simulink model "Gain_TestGen12"  (R2017b)
settings: Solver=FixedStepDiscrete  StartTime=0.0  StopTime=10.0  RelTol=1e-3
undefined symbols (not defined in the file): Block_TestLib, trigger
settings Model: Creator=ktrinh  LastModifiedBy=ktrinh
settings DebuggingCC: ParameterOverflowMsg=none

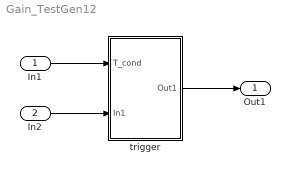
== system Gain_TestGen12 ==
  In1 : Inport
  In2 : Inport  Port=2
  trigger : Subsystem  AncestorBlock=Block_TestLib/trigger
  Out1 : Outport
  wires:
  In1/1 -> trigger/1(T_cond)
  In2/1 -> trigger/2(In1)
  trigger/1(Out1) -> Out1/1

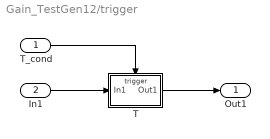
== system Gain_TestGen12/trigger ==
  T_cond : Inport  OutDataTypeStr=boolean
  In1 : Inport  Port=2
  T : Subsystem  TreatAsAtomicUnit=on
  Out1 : Outport
  wires:
  T_cond/1 -> T/Trigger
  In1/1 -> T/1(In1)
  T/1(Out1) -> Out1/1

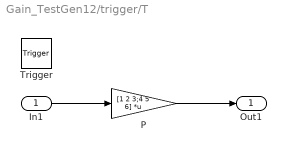
== system Gain_TestGen12/trigger/T ==
  In1 : Inport  PortDimensions=[1,3]
  Trigger : TriggerPort  VariantControl=Variant
  P : Gain  Gain=[1 2 3;4 5 6]  Multiplication=Matrix(K*u) (u vector)  OutMin=1.  OutMax=100  OutDataTypeStr=int8  RndMeth=Round  SaturateOnIntegerOverflow=on  ParamDataTypeStr=Inherit: Same as input  LockScale=on
  Out1 : Outport
  wires:
  In1/1 -> P/1
  P/1 -> Out1/1
